simulink model "WheelControl"  (R2017b)
settings: Solver=VariableStepAuto  StartTime=0.0  StopTime=inf  RelTol=1e-3
libraries: realtime_pacer_lib x1
settings Model: Creator=SYSTEM  LastModifiedBy=segadiallo
settings HardwareCC: ProdBitPerLong=64  ProdHWDeviceType=Intel->x86-64 (Mac OS X)
settings CodeAppCC: StateflowObjectComments=on

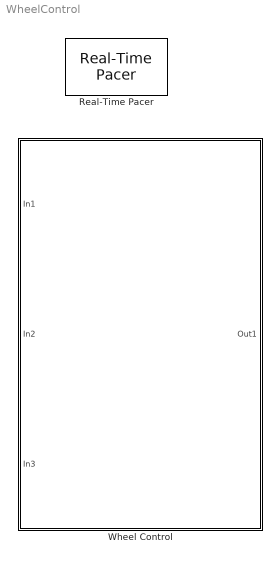
== system WheelControl ==
  Real-Time Pacer : realtime_pacer_lib/Real-Time Pacer  simTimePerRealTime=1
  Wheel Control : Subsystem
      mask help: Wheel Control
      mask Display:
      | disp('Wheel Controle');
      | port_label('output',1,'Status');
      | port_label('input',2,'rightW');
      | port_label('input',1,'InputV');
      | port_label('input',3,'leftW');

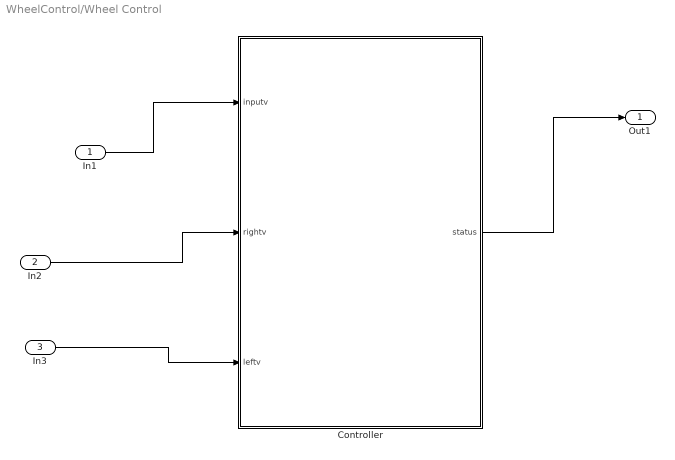
== system WheelControl/Wheel Control ==
  In1 : Inport
  In2 : Inport  Port=2
  In3 : Inport  Port=3
  Controller : Stateflow chart  TreatAsAtomicUnit=on
  Out1 : Outport
  wires:
  Controller/1(status) -> Out1/1
  In3/1 -> Controller/3(leftv)
  In2/1 -> Controller/2(rightv)
  In1/1 -> Controller/1(inputv)

== stateflow chart WheelControl/Wheel Control/Controller ==
  state NoCommand
    entry:
    status=0
  state Start
    during:
    entry:
    coder.extrinsic('evalin');
    obj = evalin('base','objWs');
    SetWheelVelRoomba(obj, rightv, leftv)
    status = 1;
  state Reset
    entry:
    coder.extrinsic('evalin');
    obj = evalin('base','objWs');
    fwrite(obj, 7)
  (default) -> NoCommand
  NoCommand -> Start : [inputv==3 ]
  Start -> Start [order 2] : after(0.1,sec)
  Start -> Reset [order 1] : [inputv==1]
  data: inputv input size=1; status output; so local; rightv input; leftv input
